simulink model "ammclib_mlib_convert_s32k14x"  (Simulink 9.0)
settings: Solver=FixedStepDiscrete  StartTime=0.0  StopTime=5  FixedStep=0.001  RelTol=1e-3  EnableMultiTasking=on
InitFcn:
  | mbd_s32k_consistency_checks(bdroot(gcs));
undefined symbols (not defined in the file): LQFP
libraries: ammclib_bam_s32k14x x12, simulink x5, mbd_s32k1xx_ec_toolbox x2
Description:
  | This model tests the AMMCLIB MLIB CONVERT blocks
  | 
  | Validation:
  | - Run the model in Simulation and compare the Inputs vs Outputs results.
  | - Open Freemaster (ammclib_mlib_convert_s32k14x.pmp) and compare the HW results against the Simulated ones
settings Model: Creator=NXP MBDT Team  LastModifiedBy=nxf35172
settings DataIOCC: ExternalInput=off  InitialState=off  LimitDataPoints=on  SaveOutput=off  SignalLogging=off  SaveTime=off
settings OptimizationCC: DefaultParameterBehavior=Inlined  LifeSpan=1
settings DebuggingCC: SolverPrmCheckMsg=warning  InheritedTsInSrcMsg=none  SingleTaskRateTransMsg=error  ParameterPrecisionLossMsg=none  UnconnectedInputMsg=error  UnconnectedOutputMsg=error  UnconnectedLineMsg=error  AllowSymbolicDim=off  UnknownTsInhSupMsg=error  StateNameClashWarn=warning
settings HardwareCC: ProdLargestAtomicInteger=Long  ProdLargestAtomicFloat=Double  ProdEndianess=LittleEndian  ProdHWDeviceType=ARM Compatible->ARM Cortex
settings SFSimCC: MATLABDynamicMemAlloc=off
settings RTWCC: SystemTargetFile=mbd_s32k.tlc  MakeCommand=mbd_s32k_make_rtw COPY_MDLREF_INCLUDES=0  TemplateMakefile=mbd_s32k.tmf  Description=Model Based Design Toolbox S32K14x Code Generation Target
settings CodeAppCC: IgnoreCustomStorageClasses=off
settings STFCustomTargetCC: CombineOutputUpdateFcns=on  ERTCustomFileBanners=on  SupportContinuousTime=off  SupportNonInlinedSFcns=off  RemoveResetFunc=on  MATLABClassNameForMDSCustomization=Simulink.SoftwareTarget.ERTCustomization  GRTInterface=off  SystemTargetFile=mbd_s32k14.tlc
settings ERTTargetCC: MultiwordLength=2048  ParMdlRefBuildCompliant=off  CompOptLevelCompliant=off  ConcurrentExecutionCompliant=off  ModelStepFunctionPrototypeControlCompliant=off  CPPClassGenCompliant=off  UseToolchainInfoCompliant=off  InlinedParameterPlacement=NonHierarchical  ERTCustomFileTemplate=example_file_process.tlc  ConvertIfToSwitch=off  SuppressUnreachableDefaultCases=off

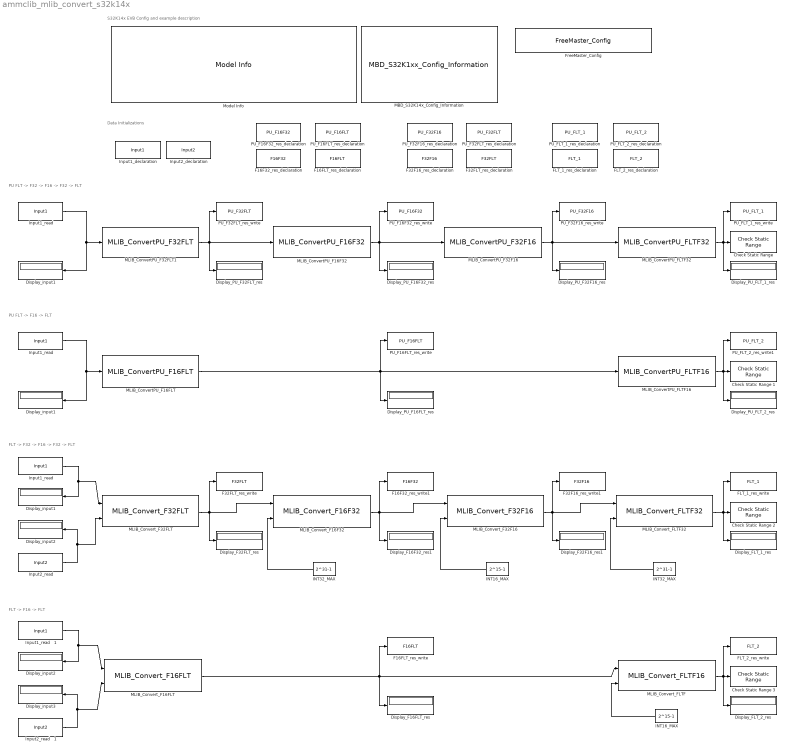
== system ammclib_mlib_convert_s32k14x ==
  note: S32K14x EVB Config and example description
  note: Data Initializations
  note: PU FLT -> F32 -> F16 -> F32 -> FLT
  note: PU FLT -> F16 -> FLT
  note: FLT -> F32 -> F16 -> F32 -> FLT
  note: FLT -> F16 -> FLT
  " Display_input1" : Display
  " Display_input2" : Display
  "Check Static Range " : simulink/Model Verification/Check  Static Range  Description=0.25 <= u <= 0.25  max=0.25  max_included=on  min=0.25  min_included=on  enabled=on  stopWhenAssertionFail=on  export=off  icon=graphic
      settings: SourceProductName=Simulink  SourceProductBaseCode=SL
  Check Static Range 1 : simulink/Model Verification/Check  Static Range  Description=0.25 <= u <= 0.25  max=0.25  max_included=on  min=0.25  min_included=on  enabled=on  stopWhenAssertionFail=on  export=off  icon=graphic
      settings: SourceProductName=Simulink  SourceProductBaseCode=SL
  Check Static Range 2 : simulink/Model Verification/Check  Static Range  Description=0.24 <= u <= 0.26  max=0.26  max_included=on  min=0.24  min_included=on  enabled=on  stopWhenAssertionFail=on  export=off  icon=graphic
      settings: SourceProductName=Simulink  SourceProductBaseCode=SL
  Check Static Range 3 : simulink/Model Verification/Check  Static Range  Description=0.24 <= u <= 0.26  max=0.26  max_included=on  min=0.24  min_included=on  enabled=on  stopWhenAssertionFail=on  export=off  icon=graphic
      settings: SourceProductName=Simulink  SourceProductBaseCode=SL
  Display_F16F32_res1 : Display
  Display_F16FLT_res : Display
  Display_F32F16_res1 : Display
  Display_F32FLT_res : Display
  Display_FLT_1_res : Display
  Display_FLT_2_res : Display
  Display_PU_F16F32_res : Display
  Display_PU_F16FLT_res : Display
  Display_PU_F32F16_res : Display
  Display_PU_F32FLT_res : Display
  Display_PU_FLT_1_res : Display
  Display_PU_FLT_2_res : Display
  Display_input1 : Display
  "Display_input1      " : Display
  Display_input2 : Display
  Display_input3 : Display
  F16F32_res_declaration : DataStoreMemory  Priority=2  DataStoreName=F16F32  ReadBeforeWriteMsg=warning  WriteAfterWriteMsg=warning  WriteAfterReadMsg=warning  ShowAdditionalParam=off  OutDataTypeStr=int16
  F16F32_res_write1 : DataStoreWrite  DataStoreName=F16F32
  F16FLT_res_declaration : DataStoreMemory  Priority=2  DataStoreName=F16FLT  ReadBeforeWriteMsg=warning  WriteAfterWriteMsg=warning  WriteAfterReadMsg=warning  ShowAdditionalParam=off  OutDataTypeStr=int16
  F16FLT_res_write : DataStoreWrite  DataStoreName=F16FLT
  F32F16_res_declaration : DataStoreMemory  Priority=2  DataStoreName=F32F16  ReadBeforeWriteMsg=warning  WriteAfterWriteMsg=warning  WriteAfterReadMsg=warning  ShowAdditionalParam=off  OutDataTypeStr=int32
  F32F16_res_write1 : DataStoreWrite  DataStoreName=F32F16
  F32FLT_res_declaration : DataStoreMemory  Priority=2  DataStoreName=F32FLT  ReadBeforeWriteMsg=warning  WriteAfterWriteMsg=warning  WriteAfterReadMsg=warning  ShowAdditionalParam=off  OutDataTypeStr=int32
  F32FLT_res_write : DataStoreWrite  DataStoreName=F32FLT
  FLT_1_res_declaration : DataStoreMemory  Priority=2  DataStoreName=FLT_1  ReadBeforeWriteMsg=warning  WriteAfterWriteMsg=warning  WriteAfterReadMsg=warning  ShowAdditionalParam=off  OutDataTypeStr=single
  FLT_1_res_write : DataStoreWrite  DataStoreName=FLT_1
  FLT_2_res_declaration : DataStoreMemory  Priority=2  DataStoreName=FLT_2  ReadBeforeWriteMsg=warning  WriteAfterWriteMsg=warning  WriteAfterReadMsg=warning  ShowAdditionalParam=off  OutDataTypeStr=single
  FLT_2_res_write : DataStoreWrite  DataStoreName=FLT_2
  FreeMaster_Config : mbd_s32k1xx_ec_toolbox/Utility Blocks/FreeMaster_Config  interface=LPUART1  baudrate=115200  rxd=PTC6: [LPUART1_RX | Receive]  txd=PTC7: [LPUART1_TX | Transmit]  mode=Short Interrupt  isr_prio=15  show_adv_opts=off  use_scope=on  max_scope_vars=8  use_recorder=on  max_rec_vars=8  rec_buff_size=1024  rec_timebase=0 milliseconds  comm_buffer_size_auto=on  comm_buffer_size=255  comm_rqueue_size_default=on  comm_rqueue_size=32
  INT16_MAX : Constant  Value=2^15-1  OutDataTypeStr=Inherit: Inherit via back propagation
  "INT16_MAX  " : Constant  Value=2^15-1  OutDataTypeStr=Inherit: Inherit via back propagation
  INT32_MAX : Constant  Value=2^31-1  OutDataTypeStr=Inherit: Inherit via back propagation
  "INT32_MAX " : Constant  Value=2^31-1  OutDataTypeStr=Inherit: Inherit via back propagation
  Input1_declaration : DataStoreMemory  Priority=1  DataStoreName=Input1  WriteAfterWriteMsg=warning  WriteAfterReadMsg=warning  InitialValue=0.25  ShowAdditionalParam=off  OutMin=-1  OutMax=1  OutDataTypeStr=single
  Input1_read : DataStoreRead  DataStoreName=Input1
  "Input1_read  " : DataStoreRead  DataStoreName=Input1
  "Input1_read   " : DataStoreRead  DataStoreName=Input1
  Input1_read   1 : DataStoreRead  DataStoreName=Input1
  Input2_declaration : DataStoreMemory  Priority=1  DataStoreName=Input2  WriteAfterWriteMsg=warning  WriteAfterReadMsg=warning  InitialValue=1  ShowAdditionalParam=off  OutMin=-1  OutMax=1  OutDataTypeStr=single
  "Input2_read   " : DataStoreRead  DataStoreName=Input2
  Input2_read   1 : DataStoreRead  DataStoreName=Input2
  MBD_S32K14x_Config_Information : mbd_s32k1xx_ec_toolbox/MBD_S32K1xx_Config_Information  Priority=0  mbdt_ver=0  disp_str=|  config_params=[]  mcu_target_name=S32K144  mcu_target_package=100-LQFP  mcu_target_sram_size=64KB  mcu_system_clock_freq=80  mcu_xtal_freq=External 8  mcu_steptick_timer=LPIT Channel 0  mcu_steptick_prio=15  ds_import_enable=on  target_compiler=GCC  target_memory=FLASH  gcc_target_compile_opts=-mcpu=cortex-m4 -mthumb -mfloat-abi=hard -mfpu=fpv4-sp-d16 -O1 -g -gstrict-dwarf  gcc_target_assemble_opts=-mcpu=cortex-m4 -mthumb -mfloat-abi=hard -mfpu=fpv4-sp-d16 -g  gcc_target_link_opts=-mcpu=cortex-m4 -mthumb -mfloat-abi=hard -mfpu=fpv4-sp-d16  gcc_target_default_lcf=on  gcc_target_user_lcf=S32K144_64_flash.ld  ghs_target_compile_opts=-cpu=cortexm4f -thumb -DARM_MATH_CM4 -fpu=vfpv4_d16 -fsingle -Ogeneral -Wundef -Wimplicit-int -Wshadow -Wtrigraphs --no_commons --gnu_asm -gnu99 -gdwarf-2 -G  ghs_target_assemble_opts=-cpu=cortexm4f -fpu=vfpv4_d16  ghs_target_link_opts=-cpu=cortexm4f -thumb -fpu=vfpv4_d16  ghs_target_default_lcf=off  ghs_target_user_lcf=S32K144_64_flash.ld  iar_target_compile_opts=--cpu=Cortex-M4F --thumb --fpu=VFPv4_sp -Ol -e --debug --dlib_config normal  iar_target_assemble_opts=--cpu Cortex-M4F --thumb --fpu VFPv4_sp  iar_target_link_opts=--no_exceptions --vfe --inline  iar_target_default_lcf=off  iar_target_user_lcf=S32K144_64_flash.icf  pil_download_enable=off  rbl_download_enable=on  rbl_start_delay=5000000  rbl_download_interface=OpenSDA  rbl_restart_request=off  rbl_com_port=Custom  rbl_com_port_custom=COM1  pil_download_rate=57600  pil_opensda_drive=Custom  pil_opensda_drive_custom=D  pil_uart_instance=0  pil_uart_rx=PTA2: [LPUART0_RX | Receive]  pil_uart_tx=PTA3: [LPUART0_TX | Transmit]  FTM_PWM_PcrCheckEnDis=on  FTM_Input_Edge_Inputs_PcrCheckEnDis=on  FTM_Dual_Edge_Inputs_PcrCheckEnDis=on  FTM_Quadrature_Inputs_PcrCheckEnDis=on  FTM_Hall_Sensor_Inputs_PcrCheckEnDis=on  LPTMR_PcrCheckEnDis=on  PIT_PcrCheckEnDis=on  RTC_PcrCheckEnDis=on  FlexCAN_PcrCheckEnDis=on  LIN_PcrCheckEnDis=on  FlexIO_PcrCheckEnDis=on  LPI2C_PcrCheckEnDis=on  LPSPI_PcrCheckEnDis=on  LPUART_PcrCheckEnDis=on  CMP_PcrCheckEnDis=on  GPIO_OutputPcrCheckEnDis=on  GPIO_InputPcrCheckEnDis=on  SBC_PcrCheckEnDis=on  AMMCLIB_PcrCheckEnDis=on  FM_PcrCheckEnDis=on  Profile_PcrCheckEnDis=on  ConfigParams_PcrCheckEnDis=on  ModelRef_PcrCheckEnDis=on  PDB0_PcrCheckEnDis=on  CSEc_PcrCheckEnDis=on  eDMA_PcrCheckEnDis=on  ADC_PcrCheckEnDis=on  WDOG_PcrCheckEnDis=on
      | Target : S32K142-16KB_SRAM
      | Package : 100-pin
      | System clock : 80 MHz
      | XTAL clock : External 8 MHz
      | Compiler : GCC
      | Target Type : FLASH
      | Download Code after build : (OpenSDA: E)
      | Step Tick Interrupt Priority : 15
  MLIB_ConvertPU_F16F32 : ammclib_bam_s32k14x/MLIB/bam_f16/MLIB_ConvertPU_F16F32
  MLIB_ConvertPU_F16FLT : ammclib_bam_s32k14x/MLIB/bam_f16/MLIB_ConvertPU_F16FLT
  MLIB_ConvertPU_F32F16 : ammclib_bam_s32k14x/MLIB/bam_f32/MLIB_ConvertPU_F32F16
  MLIB_ConvertPU_F32FLT1 : ammclib_bam_s32k14x/MLIB/bam_f32/MLIB_ConvertPU_F32FLT
  MLIB_ConvertPU_FLTF16 : ammclib_bam_s32k14x/MLIB/bam_flt/MLIB_ConvertPU_FLTF16
  MLIB_ConvertPU_FLTF32 : ammclib_bam_s32k14x/MLIB/bam_flt/MLIB_ConvertPU_FLTF32
  MLIB_Convert_F16F32 : ammclib_bam_s32k14x/MLIB/bam_f16/MLIB_Convert_F16F32
  MLIB_Convert_F16FLT : ammclib_bam_s32k14x/MLIB/bam_f16/MLIB_Convert_F16FLT
  MLIB_Convert_F32F16 : ammclib_bam_s32k14x/MLIB/bam_f32/MLIB_Convert_F32F16
  MLIB_Convert_F32FLT : ammclib_bam_s32k14x/MLIB/bam_f32/MLIB_Convert_F32FLT
  "MLIB_Convert_FLTF " : ammclib_bam_s32k14x/MLIB/bam_flt/MLIB_Convert_FLTF16
  MLIB_Convert_FLTF32 : ammclib_bam_s32k14x/MLIB/bam_flt/MLIB_Convert_FLTF32
  Model Info : simulink/Model-Wide Utilities/Model Info  Frame=off  DisplayStringWithTags=|  HorizontalTextAlignment=Left  LeftAlignmentValue=0.02
      | Model Name: %<ModelName>
      | 
      | Description: %<Description>
  PU_F16F32_res_declaration : DataStoreMemory  Priority=2  DataStoreName=PU_F16F32  ReadBeforeWriteMsg=warning  WriteAfterWriteMsg=warning  WriteAfterReadMsg=warning  ShowAdditionalParam=off  OutDataTypeStr=int16
  PU_F16F32_res_write : DataStoreWrite  DataStoreName=PU_F16F32
  PU_F16FLT_res_declaration : DataStoreMemory  Priority=2  DataStoreName=PU_F16FLT  ReadBeforeWriteMsg=warning  WriteAfterWriteMsg=warning  WriteAfterReadMsg=warning  ShowAdditionalParam=off  OutDataTypeStr=int16
  PU_F16FLT_res_write : DataStoreWrite  DataStoreName=PU_F16FLT
  PU_F32F16_res_declaration : DataStoreMemory  Priority=2  DataStoreName=PU_F32F16  ReadBeforeWriteMsg=warning  WriteAfterWriteMsg=warning  WriteAfterReadMsg=warning  ShowAdditionalParam=off  OutDataTypeStr=int32
  PU_F32F16_res_write : DataStoreWrite  DataStoreName=PU_F32F16
  PU_F32FLT_res_declaration : DataStoreMemory  Priority=2  DataStoreName=PU_F32FLT  ReadBeforeWriteMsg=warning  WriteAfterWriteMsg=warning  WriteAfterReadMsg=warning  ShowAdditionalParam=off  OutDataTypeStr=int32
  PU_F32FLT_res_write : DataStoreWrite  DataStoreName=PU_F32FLT
  PU_FLT_1_res_declaration : DataStoreMemory  Priority=2  DataStoreName=PU_FLT_1  ReadBeforeWriteMsg=warning  WriteAfterWriteMsg=warning  WriteAfterReadMsg=warning  ShowAdditionalParam=off  OutDataTypeStr=single
  PU_FLT_1_res_write : DataStoreWrite  DataStoreName=PU_FLT_1
  PU_FLT_2_res_declaration : DataStoreMemory  Priority=2  DataStoreName=PU_FLT_2  ReadBeforeWriteMsg=warning  WriteAfterWriteMsg=warning  WriteAfterReadMsg=warning  ShowAdditionalParam=off  OutDataTypeStr=single
  PU_FLT_2_res_write1 : DataStoreWrite  DataStoreName=PU_FLT_2
  wires:
  Input1_read/1 -> MLIB_ConvertPU_F32FLT1/1, Display_input1/1
  MLIB_ConvertPU_F16F32/1 -> Display_PU_F16F32_res/1, PU_F16F32_res_write/1, MLIB_ConvertPU_F32F16/1
  MLIB_ConvertPU_F32FLT1/1 -> Display_PU_F32FLT_res/1, PU_F32FLT_res_write/1, MLIB_ConvertPU_F16F32/1
  MLIB_ConvertPU_F32F16/1 -> Display_PU_F32F16_res/1, PU_F32F16_res_write/1, MLIB_ConvertPU_FLTF32/1
  MLIB_ConvertPU_FLTF32/1 -> "Check Static Range "/1, Display_PU_FLT_1_res/1, PU_FLT_1_res_write/1
  "Input1_read  "/1 -> MLIB_ConvertPU_F16FLT/1, "Display_input1      "/1
  MLIB_ConvertPU_F16FLT/1 -> MLIB_ConvertPU_FLTF16/1, PU_F16FLT_res_write/1, Display_PU_F16FLT_res/1
  MLIB_ConvertPU_FLTF16/1 -> Check Static Range 1/1, Display_PU_FLT_2_res/1, PU_FLT_2_res_write1/1
  "Input1_read   "/1 -> MLIB_Convert_F32FLT/1, " Display_input1"/1
  MLIB_Convert_F16F32/1 -> MLIB_Convert_F32F16/1, F16F32_res_write1/1, Display_F16F32_res1/1
  MLIB_Convert_F32FLT/1 -> MLIB_Convert_F16F32/1, Display_F32FLT_res/1, F32FLT_res_write/1
  MLIB_Convert_F32F16/1 -> MLIB_Convert_FLTF32/1, F32F16_res_write1/1, Display_F32F16_res1/1
  MLIB_Convert_FLTF32/1 -> Check Static Range 2/1, Display_FLT_1_res/1, FLT_1_res_write/1
  "Input2_read   "/1 -> Display_input2/1, MLIB_Convert_F32FLT/2
  INT32_MAX/1 -> MLIB_Convert_F16F32/2
  INT16_MAX/1 -> MLIB_Convert_F32F16/2
  Input1_read   1/1 -> MLIB_Convert_F16FLT/1, " Display_input2"/1
  MLIB_Convert_F16FLT/1 -> "MLIB_Convert_FLTF "/1, F16FLT_res_write/1, Display_F16FLT_res/1
  "MLIB_Convert_FLTF "/1 -> Check Static Range 3/1, Display_FLT_2_res/1, FLT_2_res_write/1
  Input2_read   1/1 -> MLIB_Convert_F16FLT/2, Display_input3/1
  "INT32_MAX "/1 -> MLIB_Convert_FLTF32/2
  "INT16_MAX  "/1 -> "MLIB_Convert_FLTF "/2
